simulink model "accel_tc_sweep_sim"  (R2026a)
settings: Solver=FixedStepDiscrete  StopTime=7  FixedStep=0.0005
PreLoadFcn:
  | addpath(fullfile(fileparts(which('params_cfr26')),'lib'));
InitFcn:
  | addpath(fullfile(fileparts(which('params_cfr26')),'lib'));
settings Model: Creator=Aboud  LastModifiedBy=Aboud

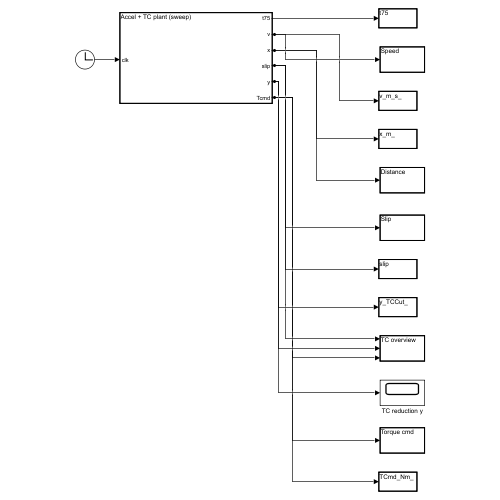
[thumbnail: Simulink's stored preview of the top-level diagram]
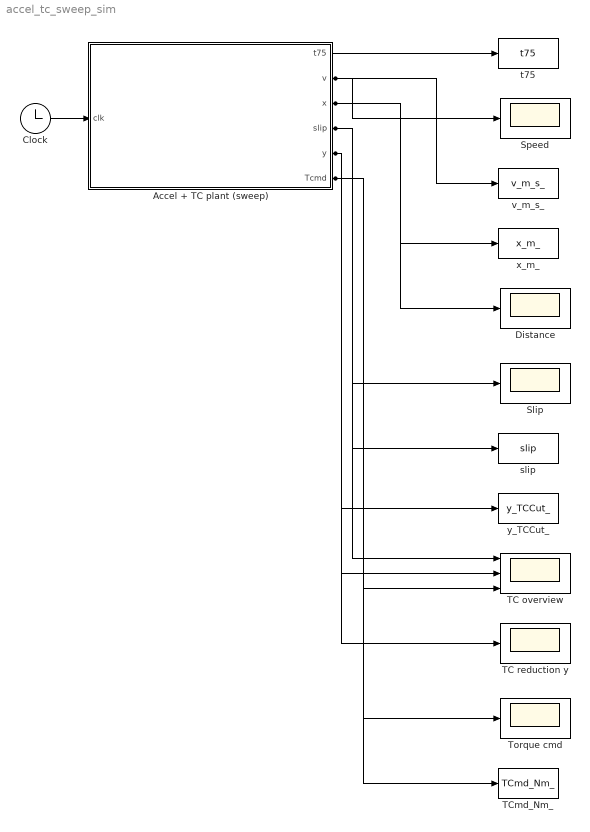
== system accel_tc_sweep_sim ==
  Accel + TC plant (sweep) : MATLAB Function  TreatAsAtomicUnit=on
  Clock : Clock
  Distance : Scope
  Slip : Scope
  Speed : Scope
  TC overview : Scope  NumInputPorts=3
  TC reduction y : Scope
  TCmd_Nm_ : ToWorkspace  VariableName=TCmd_Nm_  SaveFormat=Structure With Time  SampleTime=-1
  Torque cmd : Scope
  slip : ToWorkspace  VariableName=slip  SaveFormat=Structure With Time  SampleTime=-1
  t75 : ToWorkspace  VariableName=t75  SaveFormat=Structure With Time  SampleTime=-1
  v_m_s_ : ToWorkspace  VariableName=v_m_s_  SaveFormat=Structure With Time  SampleTime=-1
  x_m_ : ToWorkspace  VariableName=x_m_  SaveFormat=Structure With Time  SampleTime=-1
  y_TCCut_ : ToWorkspace  VariableName=y_TCCut_  SaveFormat=Structure With Time  SampleTime=-1
  wires:
  Clock/1 -> Accel + TC plant (sweep)/1(clk)
  Accel + TC plant (sweep)/3(x) -> x_m_/1, Distance/1
  Accel + TC plant (sweep)/2(v) -> v_m_s_/1, Speed/1
  Accel + TC plant (sweep)/1(t75) -> t75/1
  Accel + TC plant (sweep)/6(Tcmd) -> TCmd_Nm_/1, Torque cmd/1, TC overview/3
  Accel + TC plant (sweep)/4(slip) -> Slip/1, TC overview/1, slip/1
  Accel + TC plant (sweep)/5(y) -> y_TCCut_/1, TC reduction y/1, TC overview/2

== matlab function accel_tc_sweep_sim/Accel + TC plant (sweep) ==
  data: t75 output; v output; x output; slip output; clk input; y output; Tcmd output
function [t75, v, x, slip, y, Tcmd] = fcn(clk)
% Thin wrapper. All physics + control live in lib/accel_tc_core.m, reached
% through lib/accel_tc_sweep_sample.m, whose cache is keyed on the config so a
% sweep cannot silently reuse the previous run's trace.
coder.extrinsic('accel_tc_sweep_sample');
t75 = 0; v = 0; x = 0; slip = 0; y = 0; Tcmd = 0;
[t75, v, x, slip, y, Tcmd] = accel_tc_sweep_sample(clk);
